simulink subsystem "PieroAJModel"  (R2023b)
settings: Solver=VariableStepAuto  StartTime=0.0  StopTime=10.0  RelTol=1e-3
settings Model: Creator=Antonio  LastModifiedBy=Antonio

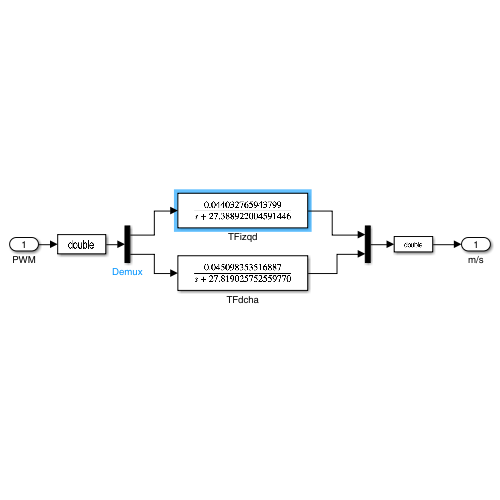
[thumbnail: Simulink's stored preview of the top-level diagram]
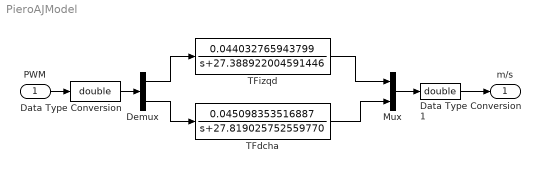
== system PieroAJModel ==
  PWM : Inport
  Data Type Conversion : DataTypeConversion  OutDataTypeStr=double  SaturateOnIntegerOverflow=off  RndMeth=Floor
  Data Type Conversion1 : DataTypeConversion  OutDataTypeStr=double  SaturateOnIntegerOverflow=off  RndMeth=Floor
  Demux : Demux  Outputs=2
  Mux : Mux  Inputs=2
  TFdcha : TransferFcn  Numerator=0.045098353516887  Denominator=[1,27.819025752559770]
  TFizqd : TransferFcn  Numerator=0.044032765943799  Denominator=[1,27.388922004591446]
  m/s : Outport
  wires:
  Demux/1 -> TFizqd/1
  Demux/2 -> TFdcha/1
  TFizqd/1 -> Mux/1
  TFdcha/1 -> Mux/2
  PWM/1 -> Data Type Conversion/1
  Data Type Conversion/1 -> Demux/1
  Mux/1 -> Data Type Conversion1/1
  Data Type Conversion1/1 -> m/s/1
